simulink library "simeventsgenerators1"  (Simulink 7.5)
settings: Solver=ode45  SolverMode=SingleTasking  StartTime=0.0  StopTime=10.0  RelTol=1e-3
undefined symbols (not defined in the file or in its folder): des_support, gcbh
libraries: des_sfun_lib x4
settings Model: Creator=mclune  LastModifiedBy=ywu  ExtModeAutoUpdateStatusClock=off
settings Model: ForwardingTableString=|
  | ||__slOldName__||simeventsgenerators1/Signal Generators/Discrete Event
  | Random Number||__slNewName__||des_test_lib/Discrete Event
  | Random Number

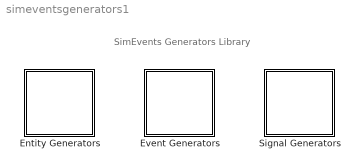
== system simeventsgenerators1 ==
  note: SimEvents Generators Library
  Entity Generators : Subsystem
      mask Type: SimEvents Sinks
      mask Display: image(imread('seGenEntity.bmp'),'center');
  Event Generators : Subsystem
      mask Type: SimEvents Sinks
      mask Display: image(imread('seGenEvent.bmp'),'center');
  Signal Generators : Subsystem
      mask Type: SimEvents Sinks
      mask Display: image(imread('seGenSignal.bmp'),'center')

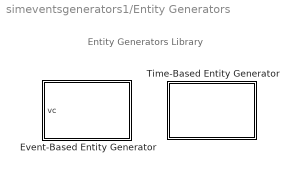
== system simeventsgenerators1/Entity Generators ==
  note: Entity Generators Library
  Event-Based Entity Generator : Subsystem  Priority=1  DialogController=des_ddg_create  DialogControllerArgs=DataTag1  LoadFcn=des_support('desLoadFcn',gcbh)  StartFcn=des_support('desStartFcn',gcbh)  StopFcn=des_support('desStopFcn',gcbh)  mask(Event-Based Entity Generator){GenerateEntitiesUpon=Change in signal from port vc, SignalEdgeType=Rising, SpecifyEventPriority=off, PriorityEntityGeneration=300, GenerateEntityAtSimulationStart=on, AllowBlocking=on, ResponseDuringBlockage=Discard generated entities, EntityType=Blank, StatNumberDeparted=Off, StatPendingEntity=Off, StatAverageIntergenerationTime=Off}
      mask prompts: GenerateEntitiesUpon "Generate entities upon:"; SignalEdgeType "Type of change in signal value:"; SpecifyEventPriority "Specify event priority for entity generation"; PriorityEntityGeneration "Generation event priority:"; GenerateEntityAtSimulationStart "Generate entity at simulation start"; AllowBlocking "Allow blocking"; ResponseDuringBlockage "Response during blockage period:"; EntityType "Entity type:"; StatNumberDeparted "Number of entities departed, #d:"; StatPendingEntity "Pending entity present in block, pe:"; StatAverageIntergenerationTime "Average intergeneration time, w:"
      mask help:
      | Generate an entity upon a signal-based event or function call.
      |
      | Use the Allow OUT port blocking and optional Response during blockage period parameters to determine how the block responds when the OUT port is blocked.
      mask init:
      | des_ddg_init(gcbh,'EventBasedEntity');
      settings: CopyFcn=des_support('desCopyFcn',gcbh)  DeleteFcn=des_support('desDeleteFcn',gcbh)  UndoDeleteFcn=des_support('desUndoDeleteFcn',gcbh)  ModelCloseFcn=des_support('desModelCloseFcn',gcbh)  PreSaveFcn=des_support('desPreSaveFcn',gcbh)  PostSaveFcn=des_support('desPostSaveFcn',gcbh)  NameChangeFcn=des_support('desNameChangeFcn',gcbh)  CloseFcn=des_support('desCloseFcn',gcbh)  ErrorFcn=des_error_redirect
      mask Help: helpview(simeventsbhelp)
      mask StyleString: popup(Sample time hit from port ts|Trigger from port tr|Change in signal from port vc|Function call from port fcn),popup(Rising|Falling|Either),checkbox,edit,checkbox,checkbox,popup(Discard generated entities|Delay first pending entity),popup(Blank|Standard),popup(Off|On|Upon stop or pause),popup(Off|On|Upon stop or pause),popup(Off|On|Upon stop or pause)
      mask TabNameString: Generation Time,Generation Time,Generation Time,Generation Time,Generation Time,Generation Time,Generation Time,Entity,Statistics,Statistics,Statistics
      mask Display:
      | image(des_iconLoad('generatorEvent.jpg'),'center');
      | port_label('input',1,'vc');
      | port_label('RConn',1,'OUT');
  Time-Based Entity Generator : Subsystem  Priority=1  DialogController=des_ddg_create  DialogControllerArgs=DataTag4  LoadFcn=des_support('desLoadFcn',gcbh)  StartFcn=des_support('desStartFcn',gcbh)  StopFcn=des_support('desStopFcn',gcbh)  mask(Time-Based Entity Generator){GenerateEntitiesUpon=Intergeneration time from dialog, Distribution=Constant, Minimum=0, Maximum=1, Mean=1, InitialSeed=12345, Period=1, PriorityEntityGeneration=300, GenerateEntityAtSimulationStart=on, ResponseWhenBlocked=Pause generation, ResponseWhenUnblocked=Immediate restart, EntityType=Blank, StatNumberDeparted=Off, StatPendingEntity=Off, StatAverageIntergenerationTime=Off}
      mask prompts: GenerateEntitiesUpon "Generate entities upon:"; InitialSeed "Initial seed:"; PriorityEntityGeneration "Generation event priority:"; GenerateEntityAtSimulationStart "Generate entity at simulation start"; ResponseWhenBlocked "Response when blocked:"; ResponseWhenUnblocked "Response when unblocked:"; EntityType "Entity type:"; StatNumberDeparted "Number of entities departed, #d:"; StatPendingEntity "Pending entity present in block, pe:"; StatAverageIntergenerationTime "Average intergeneration time, w:"
      mask help:
      | Generate entities using intergeneration times from a signal or a statistical distribution.
      |
      | Use the Response when blocked and Response when unblocked parameters to determine how the block responds when the OUT port becomes blocked and later unblocked.
      mask init:
      | des_ddg_init(gcbh,'TimeBasedEntity');
      settings: CopyFcn=des_support('desCopyFcn',gcbh)  DeleteFcn=des_support('desDeleteFcn',gcbh)  UndoDeleteFcn=des_support('desUndoDeleteFcn',gcbh)  ModelCloseFcn=des_support('desModelCloseFcn',gcbh)  PreSaveFcn=des_support('desPreSaveFcn',gcbh)  PostSaveFcn=des_support('desPostSaveFcn',gcbh)  NameChangeFcn=des_support('desNameChangeFcn',gcbh)  CloseFcn=des_support('desCloseFcn',gcbh)  ErrorFcn=des_error_redirect
      mask Help: helpview(simeventsbhelp)
      mask StyleString: popup(Intergeneration time from dialog|Intergeneration time from port t),popup(Constant|Uniform|Exponential),edit,edit,edit,edit,edit,edit,checkbox,popup(Pause generation|Error),popup(Immediate restart|Delayed restart),popup(Blank|Standard),popup(Off|On|Upon stop or pause),popup(Off|On|Upon stop or pause),popup(Off|On|Upon stop or pause)
      mask TabNameString: Generation Time,Generation Time,Generation Time,Generation Time,Generation Time,Generation Time,Generation Time,Generation Time,Generation Time,Generation Time,Generation Time,Entity,Statistics,Statistics,Statistics
      mask Display:
      | image(des_iconLoad('generatorTime.jpg'),'center');
      | port_label('RConn',1,'OUT');

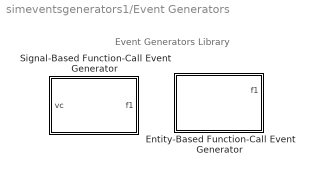
== system simeventsgenerators1/Event Generators ==
  note: Event Generators Library
  Entity-Based Function-Call Event Generator : Subsystem  Priority=1  LoadFcn=des_support('desLoadFcn',gcbh)  StartFcn=des_support('desStartFcn',gcbh)  StopFcn=des_support('desStopFcn',gcbh)  mask(Entity-Based Function-Call Event Generator){TimingFunctionCallF1=After entity departure, EnableE1Port=off, EnableF2Port=off, TimingFunctionCallF2=After entity departure, EnableE2Port=off, StatNumberDeparted=Off, StatNumberF1Calls=Off, StatNumberF2Calls=Off, IsInsideAFB=off}
      mask prompts: TimingFunctionCallF1 "Generate function call:"; EnableE1Port "Suppress function call f1 if enable signal e1 is not positive"; EnableF2Port "Generate optional function call f2 after function call f1"; TimingFunctionCallF2 "Timing of function call f2:"; EnableE2Port "Suppress function call f2 if enable signal e2  is not positive"; StatNumberDeparted "Number of entities departed, #d:"; StatNumberF1Calls "Number of f1 function calls, #f1:"; StatNumberF2Calls "Number of f2 function calls, #f2:"; IsInsideAFB "Block is inside an Attribute Function block"
      mask help: Generate a function call corresponding to each entity departure.
      mask init:
      | des_entityeventgenmask(gcb, 'init','apply')
      settings: CopyFcn=des_support('desCopyFcn',gcbh)  DeleteFcn=des_support('desDeleteFcn',gcbh)  UndoDeleteFcn=des_support('desUndoDeleteFcn',gcbh)  ModelCloseFcn=des_support('desModelCloseFcn',gcbh)  PreSaveFcn=des_support('desPreSaveFcn',gcbh)  PostSaveFcn=des_support('desPostSaveFcn',gcbh)  NameChangeFcn=des_support('desNameChangeFcn',gcbh)  CloseFcn=des_support('desCloseFcn',gcbh)
      mask Help: helpview(simeventsbhelp)
      mask StyleString: popup(Before entity departure|After entity departure),checkbox,checkbox,popup(Before entity departure|After entity departure),checkbox,popup(Off|On|Upon stop or pause),popup(Off|On|Upon stop or pause),popup(Off|On|Upon stop or pause),checkbox
      mask CallbackString: |||||des_entityeventgenmask(gcb,'cbStatNumberDeparted','noapply');|des_entityeventgenmask(gcb,'cbStatNumberF1Calls','noapply');||
      mask TabNameString: Function Call,Function Call,Function Call,Function Call,Function Call,Statistics,Statistics,Statistics,Statistics
      mask Display:
      | image(des_iconLoad('genEventEntity.jpg'),'center');
      | port_label('LConn',1,'IN');
      | port_label('RConn',1,'OUT');
      | port_label('output',1,'f1');
  Signal-Based Function-Call Event Generator : Subsystem  Priority=1  LoadFcn=des_support('desLoadFcn',gcbh)  StartFcn=des_support('desStartFcn',gcbh)  StopFcn=des_support('desStopFcn',gcbh)  mask(Signal-Based Function-Call Event Generator){GenerateFunctionCallUpon=Change in signal from port vc, SignalEdgeOption=Rising, EnableE1Port=off, EnableF2Port=off, EnableE2Port=off, SpecifyEventPriority=off, PriorityFunctionCall=200, FunctionCallDelayFrom=Dialog, DelayFunctionCall=0, StatNumberF1Calls=Off, StatNumberF2Calls=Off, MaskBlockType=none}
      mask prompts: GenerateFunctionCallUpon "Generate function call only upon:"; SignalEdgeOption "Type of change in signal value:"; EnableE1Port "Suppress function call f1 if enable signal e1 is not positive"; EnableF2Port "Generate optional f2 function call"; EnableE2Port "Suppress function call f2 if enable signal e2  is not positive"; SpecifyEventPriority "Resolve simultaneous signal updates according to event priority"; PriorityFunctionCall "Event priority:"; FunctionCallDelayFrom "Function-call delay from:"; DelayFunctionCall "Function-call time delay:"; StatNumberF1Calls "Number of f1 function calls, #f1:"; StatNumberF2Calls "Number of f2 function calls, #f2:"; MaskBlockType "Masked block type:"
      mask help:
      | Generate a function call upon each signal-based event or input function call.
      |
      | Use dialog parameters to specify the type of event that causes the block to generate a function call.
      mask init:
      | des_signaleventgenmask(gcb, 'init','apply')
      settings: CopyFcn=des_support('desCopyFcn',gcbh)  DeleteFcn=des_support('desDeleteFcn',gcbh)  UndoDeleteFcn=des_support('desUndoDeleteFcn',gcbh)  ModelCloseFcn=des_support('desModelCloseFcn',gcbh)  PreSaveFcn=des_support('desPreSaveFcn',gcbh)  PostSaveFcn=des_support('desPostSaveFcn',gcbh)  NameChangeFcn=des_support('desNameChangeFcn',gcbh)  CloseFcn=des_support('desCloseFcn',gcbh)
      mask Help: helpview(simeventsbhelp)
      mask StyleString: popup(Sample time hit from port ts|Trigger from port tr|Change in signal from port vc|Function call from port fcn),popup(Rising|Falling|Either),checkbox,checkbox,checkbox,checkbox,edit,popup(Dialog|Signal port t),edit,popup(Off|On|Upon stop or pause),popup(Off|On|Upon stop or pause),popup(none|DESS_EVENT_PORT|DESS_DATA_PORT|TOWKSPC_HAS_IC|TOWKSPC_NO_IC)
      mask CallbackString: des_signaleventgenmask(gcb,'cbFcnCallUpon','noapply');|||||des_signaleventgenmask(gcb,'cbSpecifyEventPriority','noapply');||||des_signaleventgenmask(gcb,'cbStatNumberF1Calls','noapply');||
      mask TabNameString: Function Call,Function Call,Function Call,Function Call,Function Call,Function Call,Function Call,Function Call,Function Call,Statistics,Statistics,Statistics
      mask Display:
      | image(des_iconLoad('transSigToFunc.jpg'),'center');
      | port_label('input',1,'vc');
      | port_label('output',1,'f1');

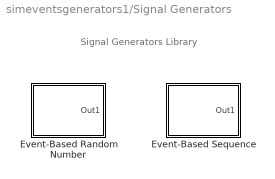
== system simeventsgenerators1/Signal Generators ==
  note: Signal Generators Library
  Event-Based Random Number : Subsystem  LoadFcn=des_support('desSfunLoadFcn',gcbh)  mask(Event-Based Random Number){distribution=Exponential, meanExp=1, minUnif=1, maxUnif=1, pOneBern=0.25, pSuccessBino=0.5, numTrialBino=1, meanNorm=0, stdNorm=1, minTri=1, maxTri=3, modeTri=2, thresholdLogn=0, scaleLogn=1, shapeLogn=1, pSuccessGeo=0.5, meanPoiss=1, thresholdLogl=0, scaleLogl=1, thresholdGam=0, scaleGam=1, shapeGam=1, minBeta=0, maxBeta=1, shape1Beta=1, shape2Beta=1, minUnid=0, maxUnid=1, numValueUnid=2, thresholdWbl=0, scaleWbl=1, shapeWbl=1, valueVecCont=[0 1], cdfVecCont=[0 1], valueVecDisc=[0 1], probVecDisc=[0.5 0.5], seed=12345, IsProcessed=on, isConnected=0}
      mask prompts: meanExp "Mean:"; minUnif "Minimum:"; maxUnif "Maximum:"; pOneBern "Probability for output to be 1:"; pSuccessBino "Probability of success in  a single trial:"; numTrialBino "Number of trials:"; meanNorm "Mean:"; stdNorm "Standard deviation:"; minTri "Minimum:"; maxTri "Maximum:"; modeTri "Mode:"; thresholdLogn "Threshold:"; scaleLogn "Mu:"; shapeLogn "Sigma:"; pSuccessGeo "Probability of success in a single trial:"; meanPoiss "Mean:"; thresholdLogl "Threshold:"; scaleLogl "Scale:"; thresholdGam "Threshold:"; scaleGam "Scale:"; shapeGam "Shape:"; minBeta "Minimum:"; maxBeta "Maximum:"; shape1Beta "Shape parameter a:"; shape2Beta "Shape parameter b:"; minUnid "Minimum:"; maxUnid "Maximum:"; numValueUnid "Number of values:"; thresholdWbl "Threshold:"; scaleWbl "Scale:"; shapeWbl "Shape:"; valueVecCont "Value vector:"; cdfVecCont "Cumulative probability function vector:"; valueVecDisc "Value vector:"; probVecDisc "Probability vector:"; seed "Initial seed:"; IsProcessed "Is Des event based signal source"; isConnected "Is Connected"
      mask help: Generate random numbers from the specified distribution, parameters, and initial seed.
      mask init:
      | des_rngsfunmask(gcb, 'init', 'apply');
      settings: CopyFcn=des_support('desSfunCopyFcn',gcbh)  NameChangeFcn=des_support('desSfunNameChangeFcn',gcbh)
      mask Help: helpview(simeventsbhelp)
      mask StyleString: popup(Exponential|Uniform|Bernoulli|Binomial|Triangular|Gamma|Gaussian (normal)|Geometric|Poisson|Lognormal|Log-logistic|Beta|Discrete uniform|Weibull|Arbitrary continuous|Arbitrary discrete),edit,edit,edit,edit,edit,edit,edit,edit,edit,edit,edit,edit,edit,edit,edit,edit,edit,edit,edit,edit,edit,edit,edit,edit,edit,edit,edit,edit,edit,edit,edit,edit,edit,edit,edit,edit,checkbox,edit
      mask CallbackString: des_rngsfunmask(gcb,'cbDistType','noapply');||||||||||||||||||||||||||||||||||||||
      mask Display: plot(0,0,100,100,[95 5 10 10 10 (100-15)*[0:1/30:1]+10],[75 75 75 70 95 70    58 76 77 63 86 86 74 78 76 73 82 69 96 73 76 85 75 74 66 77 61 82 91 68    83 87 59 60 80 71]);
  Event-Based Sequence : Subsystem  LoadFcn=des_support('desSfunLoadFcn',gcbh)  mask(Event-Based Sequence){VectorOutputValues=[3 1 4 2 1 7 5 2].', FormOutputOpt=Cyclic repetition, IsProcessed=on, isConnected=0}
      mask prompts: VectorOutputValues "Vector of output values:"; FormOutputOpt "Form output after final data value by:"; IsProcessed "Is Des event based signal source"; isConnected "Is Connected"
      mask help: Generate sequence of numbers from the specified column vector.
      mask init:
      | des_seqgen_sfunmask(gcb, 'init', 'apply');
      | try
      |     if length(VectorOutputValues) > 1000
      |         downSize = 1000; 
      |     else
      |         downSize = length(VectorOutputValues);
      |     end
      |     xval = [1 1 1 reshape([2:downSize;2:downSize],1,2*(downSize-1)) downSize+1];
      |     yval = [(min(VectorOutputValues(1:downSize))+max(VectorOutputValues(1:downSize)))/2+0.75*(max(VectorOutputValues(1:downSize))-min(VectorOutputValues(1:downSize))) (min(VectorOutputValues(1:downSize))+max(VectorOutputValues(1:downSize)))/2-0.75*(max(VectorOutputValues(1:downSize))-min(VectorOutputValues(1:downSize))) reshape([reshape(VectorOutputValues(1:downSize),1,downSize);reshape(VectorOutputValues(1:downSize),1,downSize)],1,2*downSize)];
      | catch 
      |     xval = [1 1 reshape([1:1000;2:1001],1,2000)];
      |     yval = [1249.7 -248.8 reshape([1:1000;1:1000],1,2000)];
      | end
      settings: CopyFcn=des_support('desSfunCopyFcn',gcbh)  NameChangeFcn=des_support('desSfunNameChangeFcn',gcbh)
      mask Help: helpview(simeventsbhelp)
      mask StyleString: edit,popup(Cyclic repetition|Holding final value|Setting to infinity|Setting to zero),popup(on),edit
      mask CallbackString: |des_seqgen_sfunmask(gcb,'cbFormOutput','noapply');||
      mask Display: plot(xval,yval);

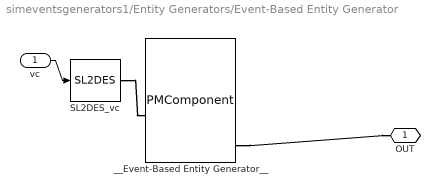
== system simeventsgenerators1/Entity Generators/Event-Based Entity Generator ==
  vc : Inport  OutDataType=sfix(16)  OutScaling=2^0
  SL2DES_vc : des_sfun_lib/SL2DES  SystemSampleTime=-1  PortType=desPortOut  PhysicalDomain=simevents  SubClassName=DES_SL2DES  timingControl=Simulink  execIndex=300  trigger=None  filter=0  updateBeforeRead=off  InitValue=0  initToFactVal=off  sampleTime=-1  offsetTime=0  idxBlockMR=0  IsMonitorOnly=off  dimsInfo=1
  __Event-Based Entity Generator__ : PMComponent  PhysicalDomain=simevents  SubClassName=DES_EVENT_BASED_ENTITYGEN  LeftPortType=desPortIn  RightPortType=desPortOut  LConnTagsString=DI|DI|DI|DI  RConnTagsString=DO|DO|DO|DO
      mask Display:
      | port_label('LConn',1,'ts');
      | port_label('LConn',2,'tr');
      | port_label('LConn',3,'vc');
      | port_label('LConn',4,'fcn');
      | port_label('RConn',1,'#d');
      | port_label('RConn',2,'pe');
      | port_label('RConn',3,'w');
      | port_label('RConn',4,'OUT');
  OUT : PMIOPort  Port=1  Side=Right
  wires:
  vc/1 -> SL2DES_vc/1
  connections:
  __Event-Based Entity Generator__/RConn4 -- OUT/RConn1
  SL2DES_vc/RConn1 -- __Event-Based Entity Generator__/LConn3

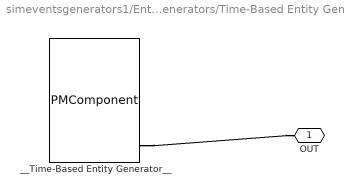
== system simeventsgenerators1/Entity Generators/Time-Based Entity Generator ==
  __Time-Based Entity Generator__ : PMComponent  PhysicalDomain=simevents  SubClassName=DES_TIME_BASED_ENTITYGEN  LeftPortType=desPortIn  RightPortType=desPortOut  LConnTagsString=DI  RConnTagsString=DO|DO|DO|DO
      mask Display:
      | port_label('LConn',1,'t');
      | port_label('RConn',1,'#d');
      | port_label('RConn',2,'pe');
      | port_label('RConn',3,'w');
      | port_label('RConn',4,'OUT');
  OUT : PMIOPort  Port=1  Side=Right
  connections:
  __Time-Based Entity Generator__/RConn4 -- OUT/RConn1

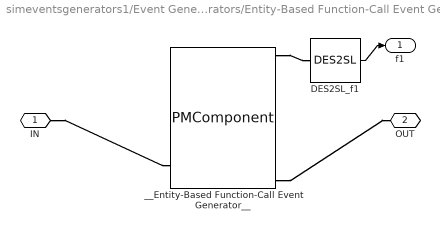
== system simeventsgenerators1/Event Generators/Entity-Based Function-Call Event Generator ==
  DES2SL_f1 : des_sfun_lib/DES2SL  SystemSampleTime=-1  PortType=desPortIn  PhysicalDomain=simevents  SubClassName=DES_DES2SL  timingControl=FunctionCall  execIndex=0  multipleOutputs=off  updateBeforeRead=off  InitValue=0  sampleTime=-1  offsetTime=0  idxBlockMR=0  IsMonitorOnly=off  dimsInfo=1
  __Entity-Based Function-Call Event Generator__ : PMComponent  PhysicalDomain=simevents  SubClassName=DES_ENTITYFUNCTIONCALL  LeftPortType=desPortIn  RightPortType=desPortOut  LConnTagsString=DI|DI|DI  RConnTagsString=DO|DO|DO|DO|DO|DO
      mask Display:
      | port_label('LConn',1,'e1');
      | port_label('LConn',2,'e2');
      | port_label('LConn',3,'IN');
      | port_label('RConn',1,'f1');
      | port_label('RConn',2,'f2');
      | port_label('RConn',3,'#d');
      | port_label('RConn',4,'#f1');
      | port_label('RConn',5,'#f2');
      | port_label('RConn',6,'OUT');
  IN : PMIOPort  Port=1  Side=Left
  OUT : PMIOPort  Port=2  Side=Right
  f1 : Outport  OutDataType=sfix(16)  OutScaling=2^0
  wires:
  DES2SL_f1/1 -> f1/1
  connections:
  IN/RConn1 -- __Entity-Based Function-Call Event Generator__/LConn3
  __Entity-Based Function-Call Event Generator__/RConn6 -- OUT/RConn1
  __Entity-Based Function-Call Event Generator__/RConn1 -- DES2SL_f1/LConn1

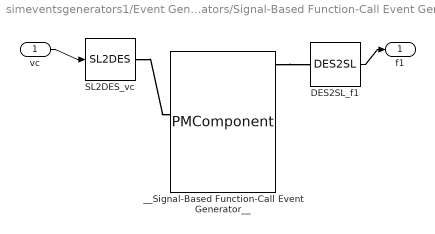
== system simeventsgenerators1/Event Generators/Signal-Based Function-Call Event Generator ==
  vc : Inport  PortDimensions=1  DataType=double  OutDataType=sfix(16)  OutScaling=2^0  OutDataTypeStr=double
  DES2SL_f1 : des_sfun_lib/DES2SL  SystemSampleTime=-1  PortType=desPortIn  PhysicalDomain=simevents  SubClassName=DES_DES2SL  timingControl=FunctionCall  execIndex=0  multipleOutputs=off  updateBeforeRead=off  InitValue=0  sampleTime=-1  offsetTime=0  idxBlockMR=0  IsMonitorOnly=off  dimsInfo=1
  SL2DES_vc : des_sfun_lib/SL2DES  SystemSampleTime=-1  PortType=desPortOut  PhysicalDomain=simevents  SubClassName=DES_SL2DES  timingControl=Simulink  execIndex=200  trigger=None  filter=0  updateBeforeRead=off  InitValue=0  initToFactVal=off  sampleTime=-1  offsetTime=0  idxBlockMR=0  IsMonitorOnly=off  dimsInfo=1
  __Signal-Based Function-Call Event Generator__ : PMComponent  PhysicalDomain=simevents  SubClassName=DES_FUNCTIONCALL  LeftPortType=desPortIn  RightPortType=desPortOut  LConnTagsString=DI|DI|DI|DI|DI|DI|DI|DI  RConnTagsString=DO|DO|DO|DO|DO
      mask Display:
      | port_label('LConn',1,'t');
      | port_label('LConn',2,'ts');
      | port_label('LConn',3,'tr');
      | port_label('LConn',4,'vc');
      | port_label('LConn',5,'fcn');
      | port_label('LConn',6,'e1');
      | port_label('LConn',7,'e2');
      | port_label('LConn',8,'IN');
      | port_label('RConn',1,'f1');
      | port_label('RConn',2,'f2');
      | port_label('RConn',3,'#f1');
      | port_label('RConn',4,'#f2');
      | port_label('RConn',5,'OUT');
  f1 : Outport  OutDataType=sfix(16)  OutScaling=2^0
  wires:
  DES2SL_f1/1 -> f1/1
  vc/1 -> SL2DES_vc/1
  connections:
  __Signal-Based Function-Call Event Generator__/RConn1 -- DES2SL_f1/LConn1
  SL2DES_vc/RConn1 -- __Signal-Based Function-Call Event Generator__/LConn4

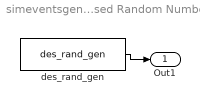
== system simeventsgenerators1/Signal Generators/Event-Based Random Number ==
  des_rand_gen : S-Function  FunctionName=des_rand_gen  Parameters="distribution, -1, seed, meanExp, minUnif, maxUnif, pOneBern, pSuccessBino, numTrialBino, meanNorm, stdNorm, minTri, maxTri, modeTri, thresholdLogn, scaleLogn, shapeLogn, pSuccessGeo, meanPoiss, thresholdLogl, scaleLogl, thresholdGam, scaleGam, shapeGam, minBeta, maxBeta, shape1Beta, shape2Beta, minUnid, maxUnid, numValueUnid, thresholdWbl, scaleWbl, shapeWbl, valueVecCont, cdfVecCont, valueVecDisc, probVecDisc,  0, 'on',isConnected"  EnableBusSupport=off  mask{IsProcessed=on}
      mask prompts: IsProcessed "DesCecSrcFlag"
  Out1 : Outport  OutDataType=sfix(16)  OutScaling=2^0
  wires:
  des_rand_gen/1 -> Out1/1

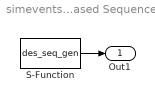
== system simeventsgenerators1/Signal Generators/Event-Based Sequence ==
  S-Function : S-Function  FunctionName=des_seq_gen  Parameters=VectorOutputValues, FormOutputOpt,IsProcessed,isConnected  EnableBusSupport=off  mask{isProcessed=on}
  Out1 : Outport  OutDataType=sfix(16)  OutScaling=2^0
  wires:
  S-Function/1 -> Out1/1
